simulink model "PX4_PID"  (R2023b)
settings: Solver=FixedStepAuto  StartTime=0.0  StopTime=inf  RelTol=1e-3  EnableMultiTasking=on
undefined symbols (not defined in the file): AUX, dev, pwm_output1
libraries: slpidlib x3, px4uORBlib x3, px4Sensorslib x2, px4lib x1, robotcorelib x1
settings Model: ExtModeTrigDuration=10  Creator=yamak  LastModifiedBy=sekiguchi
settings SolverCC: PositivePriorityOrder=on
settings OptimizationCC: EnhancedBackFolding=on  PassReuseOutputArgsAs=Individual arguments  ZeroExternalMemoryAtStartup=off  ZeroInternalMemoryAtStartup=off  MaxStackSize=64  OptimizeBlockOrder=speed  DifferentSizesBufferReuse=on  OptimizationCustomize=off  EfficientTunableParamExpr=on
settings DebuggingCC: ParameterTunabilityLossMsg=error
settings HardwareCC: ProdBitPerPointer=32  ProdBitPerSizeT=32  ProdBitPerPtrDiffT=32  ProdLargestAtomicInteger=Long  ProdLargestAtomicFloat=Double  ProdWordSize=32  ProdLongLongMode=on  ProdHWDeviceType=ARM Compatible->ARM Cortex
settings SFSimCC: MATLABDynamicMemAlloc=off  SimTargetLang=C++
settings RTWCC: Description=Embedded Coder  SystemTargetFile=ert.tlc  HardwareBoard=PX4 Pixhawk 6x  TLCOptions="-aInlineSetEventsForThisBaseRateFcn=TLC_FALSE -aSuppressMultiTaskScheduler=TLC_FALSE  -aRateBasedStepFcn=0"  TemplateMakefile=ert_default_tmf  Toolchain=GNU Tools for PX4 Autopilots  TargetLang=C++
settings CodeAppCC: ForceParamTrailComments=on  IgnoreCustomStorageClasses=off  OperatorAnnotations=on  SimulinkDataObjDesc=on  SFDataObjDesc=on  InsertBlockDesc=on
settings ERTTargetCC: ExtModeTransport=3  ExtModeStaticAlloc=on  ExtModeStaticAllocSize=1024  ExtModeMexFile=ext_xcp  ExtModeIntrfLevel=Level2 - Open

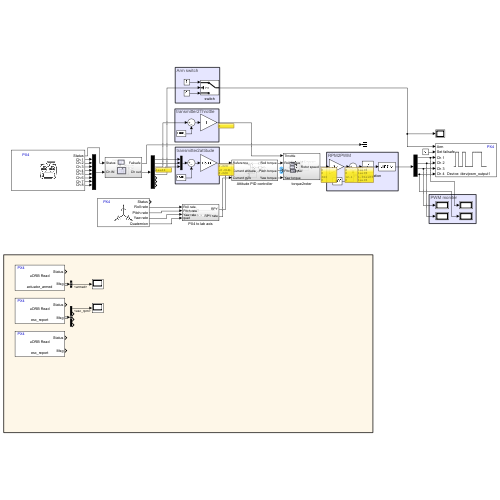
[thumbnail: Simulink's stored preview of the top-level diagram]
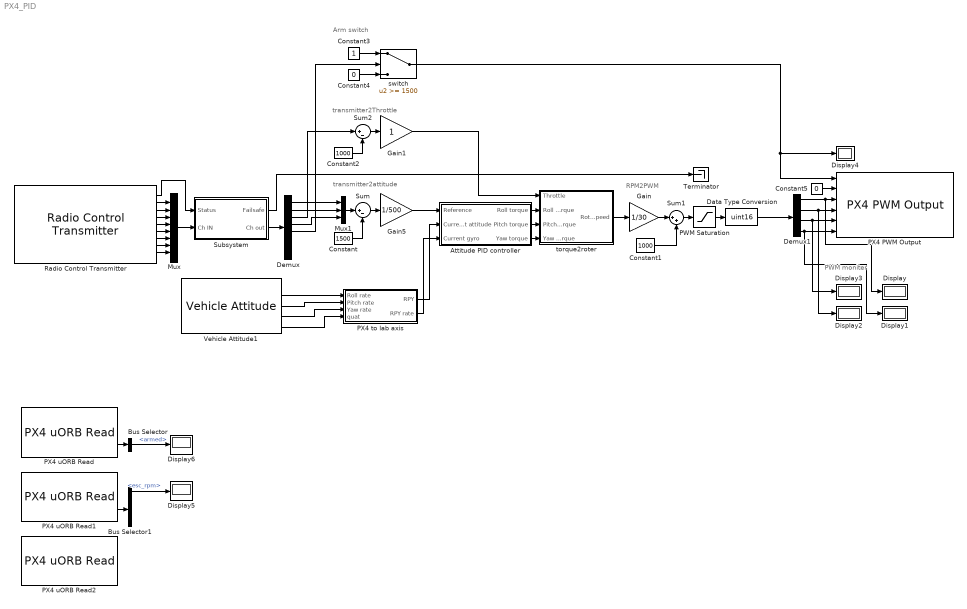
== system PX4_PID ==
  note: PWM moniter
  note: Arm switch
  note: transmitter2Throttle
  note: transmitter2attitude
  note: RPM2PWM
  Attitude PID controller : Subsystem
  Bus Selector : BusSelector  OutputSignals=armed
  Bus Selector1 : BusSelector  OutputSignals=esc_rpm,esc_voltage,esc_current,esc_temperature
  Constant : Constant  Value=1500
  Constant1 : Constant  Value=1000
  Constant2 : Constant  Value=1000
  Constant3 : Constant  OutDataTypeStr=boolean
  Constant4 : Constant  Value=0  OutDataTypeStr=boolean
  Constant5 : Constant  Value=0  OutDataTypeStr=boolean
  Data Type Conversion : DataTypeConversion  OutDataTypeStr=uint16  SaturateOnIntegerOverflow=off  RndMeth=Floor
  Demux : Demux  Outputs=8
  Demux1 : Demux
  Display{,1..6} (7 alike) : Display
  Gain : Gain  Gain=1/30
  Gain1 : Gain  OutDataTypeStr=double
  Gain5 : Gain  Gain=1/500  OutDataTypeStr=double
  Mux : Mux  Inputs=8
  Mux1 : Mux  Inputs=3
  PWM Saturation : Saturate  UpperLimit=2000  LowerLimit=1000
  PX4 PWM Output : px4lib/PX4 PWM Output  pwmDevice=AUX (/dev/pwm_output1)  pwmChannel1_=on  pwmChannel2_=on  pwmChannel3_=on  pwmChannel4_=on  pwmChannel5_=off  pwmChannel6_=off  pwmChannel7_=off  pwmChannel8_=off  forceTerminateFailsafe=off  outputErrorStatus=off
  PX4 to lab axis : Subsystem
  PX4 uORB Read : px4uORBlib/PX4 uORB Read  uORBTopic=actuator_armed  selectInstance=actuator_armed  SampleTime=0.001  BlockingMode=off  BlockTimeout=1e-3
  PX4 uORB Read1 : px4uORBlib/PX4 uORB Read  uORBTopic=esc_report  selectInstance=esc_report  SampleTime=0.001  BlockingMode=off  BlockTimeout=1e-3
  PX4 uORB Read2 : px4uORBlib/PX4 uORB Read  uORBTopic=esc_report  selectInstance=esc_report  SampleTime=0.001  BlockingMode=off  BlockTimeout=1e-3
  Radio Control Transmitter : px4Sensorslib/Radio Control Transmitter  channel1=on  channel2=on  channel3=on  channel4=on  channel5=on  channel6=on  channel7=on  channel8=on  channel_count=off  rssi=off  rc_input_source=off  timestamp_last_signal=off  time_stamp=off  sampleTime=1/250  BlockingMode=off  BlockTimeout=5
  Subsystem : Subsystem
  Sum : Sum  Inputs=|+-
  Sum1 : Sum  Inputs=|++
  Sum2 : Sum  Inputs=|+-
  Terminator : Terminator
  Vehicle Attitude1 : px4Sensorslib/Vehicle Attitude  rollRate=on  pitchRate=on  yawRate=on  quaternion=on  uorbTimeStamp=off  BlockingMode=off  BlockTimeout=0.001  sampleTime=1/250
  switch : Switch  Threshold=1500  OutDataTypeStr=boolean  SaturateOnIntegerOverflow=off  InputSameDT=off
  torque2roter : Subsystem
  wires:
  Vehicle Attitude1/5 -> PX4 to lab axis/4(quat)
  Constant/1 -> Sum/2
  Mux1/1 -> Sum/1
  Sum/1 -> Gain5/1
  Gain5/1 -> Attitude PID controller/1(Reference)
  Demux1/1 -> Display/1, PX4 PWM Output/3
  Demux1/2 -> PX4 PWM Output/4, Display2/1
  Demux1/3 -> PX4 PWM Output/5, Display3/1
  Demux1/4 -> Display1/1, PX4 PWM Output/6
  Data Type Conversion/1 -> Demux1/1
  Vehicle Attitude1/2 -> PX4 to lab axis/1(Roll rate)
  Vehicle Attitude1/3 -> PX4 to lab axis/2(Pitch rate)
  Vehicle Attitude1/4 -> PX4 to lab axis/3(Yaw rate)
  PWM Saturation/1 -> Data Type Conversion/1
  Sum1/1 -> PWM Saturation/1
  Constant1/1 -> Sum1/2
  Gain/1 -> Sum1/1
  torque2roter/1(Rotor speed) -> Gain/1
  PX4 to lab axis/1(RPY) -> Attitude PID controller/2(Current attitude)
  PX4 to lab axis/2(RPY rate) -> Attitude PID controller/3(Current gyro)
  Attitude PID controller/1(Roll torque) -> torque2roter/2(Roll torque)
  Attitude PID controller/2(Pitch torque) -> torque2roter/3(Pitch torque)
  Attitude PID controller/3(Yaw torque) -> torque2roter/4(Yaw torque)
  Sum2/1 -> Gain1/1
  Constant2/1 -> Sum2/2
  Gain1/1 -> torque2roter/1(Throttle)
  Radio Control Transmitter/1 -> Subsystem/1(Status)
  Radio Control Transmitter/9 -> Mux/8
  Radio Control Transmitter/2 -> Mux/1
  Radio Control Transmitter/3 -> Mux/2
  Radio Control Transmitter/4 -> Mux/3
  Radio Control Transmitter/5 -> Mux/4
  Radio Control Transmitter/6 -> Mux/5
  Radio Control Transmitter/7 -> Mux/6
  Radio Control Transmitter/8 -> Mux/7
  Mux/1 -> Subsystem/2(Ch IN)
  Subsystem/2(Ch out) -> Demux/1
  Demux/1 -> Mux1/1
  Demux/2 -> Mux1/2
  Demux/4 -> Mux1/3
  Demux/3 -> Sum2/1
  Constant3/1 -> switch/1
  Demux/5 -> switch/2
  Constant4/1 -> switch/3
  PX4 uORB Read/2 -> Bus Selector/1
  Bus Selector/1 -> Display6/1  "<armed>"
  switch/1 -> PX4 PWM Output/1, Display4/1
  Subsystem/1(Failsafe) -> Terminator/1
  PX4 uORB Read1/2 -> Bus Selector1/1
  Bus Selector1/1 -> Display5/1  "<esc_rpm>"
  Constant5/1 -> PX4 PWM Output/2

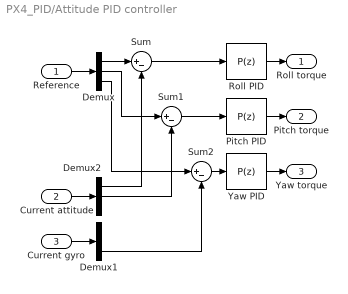
== system PX4_PID/Attitude PID controller ==
  Reference : Inport
  Current attitude : Inport  Port=2
  Current gyro : Inport  Port=3
  Demux : Demux  Outputs=3
  Demux1 : Demux  Outputs=3
  Demux2 : Demux  Outputs=3
  Pitch PID : slpidlib/PID Controller  Controller=P  Form=Parallel  TimeDomain=Discrete-time  UseExternalTs=off  SampleTime=-1  IntegratorMethod=Forward Euler  FilterMethod=Forward Euler  ControllerParametersSource=internal  P=1  I=1  UseKiTs=off  D=0  N=100  UseFilter=on  TunerSelectOption=Transfer Function Based (PID Tuner App)  InitialConditionSource=internal  InitialConditionForIntegrator=0  InitialConditionForFilter=0  DifferentiatorICPrevScaledInput=0  ExternalReset=none  TrackingMode=off  Kt=1  LimitOutput=off  SatLimitsSource=internal  UpperSaturationLimit=inf  LowerSaturationLimit=-inf  LinearizeAsGain=on  AntiWindupMode=none  Kb=1  LimitIntegrator=off  UpperIntegratorSaturationLimit=inf  LowerIntegratorSaturationLimit=-inf  POutMin=[]  POutMax=[]  IOutMin=[]  IOutMax=[]  DOutMin=[]  DOutMax=[]  NOutMin=[]  NOutMax=[]  SumOutMin=[]  SumOutMax=[]  SaturationOutMin=[]  SaturationOutMax=[]  PParamMin=[]  PParamMax=[]  IParamMin=[]  IParamMax=[]  DParamMin=[]  DParamMax=[]  NParamMin=[]  NParamMax=[]  KbParamMin=[]  KbParamMax=[]  KtParamMin=[]  KtParamMax=[]  KbOutMin=[]  KbOutMax=[]  KtOutMin=[]  KtOutMax=[]  IntegratorOutMin=[]  IntegratorOutMax=[]  FilterOutMin=[]  FilterOutMax=[]  SumI1OutMin=[]  SumI1OutMax=[]  SumI2OutMin=[]  SumI2OutMax=[]  SumI3OutMin=[]  SumI3OutMax=[]  SumI4OutMin=[]  SumI4OutMax=[]  SumDOutMin=[]  SumDOutMax=[]  DifferentiatorOutMin=[]  DifferentiatorOutMax=[]  FilterDiffOutCoefMin=[]  FilterDiffOutCoefMax=[]  ReciprocalOutMin=[]  ReciprocalOutMax=[]  SumDenOutMin=[]  SumDenOutMax=[]  SumNumOutMin=[]  SumNumOutMax=[]  DivideOutMin=[]  DivideOutMax=[]  UdiffTsProdOutMin=[]  UdiffTsProdOutMax=[]  NTsProdOutMin=[]  NTsProdOutMax=[]  UintegralTsProdOutMin=[]  UintegralTsProdOutMax=[]  UngainTsProdOutMin=[]  UngainTsProdOutMax=[]  ClampingZeroOutDataTypeStr=Inherit: Inherit via back propagation  ClampingZeroOutMin=[]  ClampingZeroOutMax=[]  FilterDenConstantOutDataTypeStr=Inherit: Inherit via back propagation  FilterDenConstantOutMin=[]  FilterDenConstantOutMax=[]  PCopyOutDataTypeStr=Inherit: Inherit via back propagation  PCopyOutMin=[]  PCopyOutMax=[]  NCopyOutDataTypeStr=Inherit: Inherit via back propagation  NCopyOutMin=[]  NCopyOutMax=[]  IntegratorContinuousStateAttributes=''  IntegratorStateMustResolveToSignalObject=off  IntegratorRTWStateStorageClass=Auto  FilterContinuousStateAttributes=''  FilterStateMustResolveToSignalObject=off  FilterRTWStateStorageClass=Auto  ParallelPVariant=InternalParameters  IdealPVariant=Disabled  IVariant=Disabled  DVariant=Disabled  IntegratorVariant=Disabled  SatVariant=Disabled  AWVariant=Disabled  PCopyVariant=Disabled  TRVariant=Disabled  FdbkBlocksVariant=Forward  IdealPFdbkVariant=Disabled  SatFdbkVariant=Disabled  DerivativeFilterVariant=Disabled  NVariant=Disabled  NCopyVariant=Disabled_SignalSpec  FilterICVariant=Disabled  IntegratorICVariant=Disabled  ExternalResetVariant=Disabled  TRSumVariant=Passthrough  SumFdbkVariant=Disabled  SumVariant=Passthrough_P  TsampFilterVariant=InternalTs  TsampNgainVariant=Passthrough  TsampIntegralVariant=Disabled_SignalSpec  ExternalSaturationOutDataTypeStr=Inherit: Same as second input
  Roll PID : slpidlib/PID Controller  Controller=P  Form=Parallel  TimeDomain=Discrete-time  UseExternalTs=off  SampleTime=-1  IntegratorMethod=Forward Euler  FilterMethod=Forward Euler  ControllerParametersSource=internal  P=1  I=1  UseKiTs=off  D=0  N=100  UseFilter=on  TunerSelectOption=Transfer Function Based (PID Tuner App)  InitialConditionSource=internal  InitialConditionForIntegrator=0  InitialConditionForFilter=0  DifferentiatorICPrevScaledInput=0  ExternalReset=none  TrackingMode=off  Kt=1  LimitOutput=off  SatLimitsSource=internal  UpperSaturationLimit=inf  LowerSaturationLimit=-inf  LinearizeAsGain=on  AntiWindupMode=none  Kb=1  LimitIntegrator=off  UpperIntegratorSaturationLimit=inf  LowerIntegratorSaturationLimit=-inf  POutMin=[]  POutMax=[]  IOutMin=[]  IOutMax=[]  DOutMin=[]  DOutMax=[]  NOutMin=[]  NOutMax=[]  SumOutMin=[]  SumOutMax=[]  SaturationOutMin=[]  SaturationOutMax=[]  PParamMin=[]  PParamMax=[]  IParamMin=[]  IParamMax=[]  DParamMin=[]  DParamMax=[]  NParamMin=[]  NParamMax=[]  KbParamMin=[]  KbParamMax=[]  KtParamMin=[]  KtParamMax=[]  KbOutMin=[]  KbOutMax=[]  KtOutMin=[]  KtOutMax=[]  IntegratorOutMin=[]  IntegratorOutMax=[]  FilterOutMin=[]  FilterOutMax=[]  SumI1OutMin=[]  SumI1OutMax=[]  SumI2OutMin=[]  SumI2OutMax=[]  SumI3OutMin=[]  SumI3OutMax=[]  SumI4OutMin=[]  SumI4OutMax=[]  SumDOutMin=[]  SumDOutMax=[]  DifferentiatorOutMin=[]  DifferentiatorOutMax=[]  FilterDiffOutCoefMin=[]  FilterDiffOutCoefMax=[]  ReciprocalOutMin=[]  ReciprocalOutMax=[]  SumDenOutMin=[]  SumDenOutMax=[]  SumNumOutMin=[]  SumNumOutMax=[]  DivideOutMin=[]  DivideOutMax=[]  UdiffTsProdOutMin=[]  UdiffTsProdOutMax=[]  NTsProdOutMin=[]  NTsProdOutMax=[]  UintegralTsProdOutMin=[]  UintegralTsProdOutMax=[]  UngainTsProdOutMin=[]  UngainTsProdOutMax=[]  ClampingZeroOutDataTypeStr=Inherit: Inherit via back propagation  ClampingZeroOutMin=[]  ClampingZeroOutMax=[]  FilterDenConstantOutDataTypeStr=Inherit: Inherit via back propagation  FilterDenConstantOutMin=[]  FilterDenConstantOutMax=[]  PCopyOutDataTypeStr=Inherit: Inherit via back propagation  PCopyOutMin=[]  PCopyOutMax=[]  NCopyOutDataTypeStr=Inherit: Inherit via back propagation  NCopyOutMin=[]  NCopyOutMax=[]  IntegratorContinuousStateAttributes=''  IntegratorStateMustResolveToSignalObject=off  IntegratorRTWStateStorageClass=Auto  FilterContinuousStateAttributes=''  FilterStateMustResolveToSignalObject=off  FilterRTWStateStorageClass=Auto  ParallelPVariant=InternalParameters  IdealPVariant=Disabled  IVariant=Disabled  DVariant=Disabled  IntegratorVariant=Disabled  SatVariant=Disabled  AWVariant=Disabled  PCopyVariant=Disabled  TRVariant=Disabled  FdbkBlocksVariant=Forward  IdealPFdbkVariant=Disabled  SatFdbkVariant=Disabled  DerivativeFilterVariant=Disabled  NVariant=Disabled  NCopyVariant=Disabled_SignalSpec  FilterICVariant=Disabled  IntegratorICVariant=Disabled  ExternalResetVariant=Disabled  TRSumVariant=Passthrough  SumFdbkVariant=Disabled  SumVariant=Passthrough_P  TsampFilterVariant=InternalTs  TsampNgainVariant=Passthrough  TsampIntegralVariant=Disabled_SignalSpec  ExternalSaturationOutDataTypeStr=Inherit: Same as second input
  Sum : Sum  Inputs=|+-
  Sum1 : Sum  Inputs=|+-
  Sum2 : Sum  Inputs=|+-
  Yaw PID : slpidlib/PID Controller  Controller=P  Form=Parallel  TimeDomain=Discrete-time  UseExternalTs=off  SampleTime=-1  IntegratorMethod=Forward Euler  FilterMethod=Forward Euler  ControllerParametersSource=internal  P=1  I=1  UseKiTs=off  D=0  N=100  UseFilter=on  TunerSelectOption=Transfer Function Based (PID Tuner App)  InitialConditionSource=internal  InitialConditionForIntegrator=0  InitialConditionForFilter=0  DifferentiatorICPrevScaledInput=0  ExternalReset=none  TrackingMode=off  Kt=1  LimitOutput=off  SatLimitsSource=internal  UpperSaturationLimit=inf  LowerSaturationLimit=-inf  LinearizeAsGain=on  AntiWindupMode=none  Kb=1  LimitIntegrator=off  UpperIntegratorSaturationLimit=inf  LowerIntegratorSaturationLimit=-inf  POutMin=[]  POutMax=[]  IOutMin=[]  IOutMax=[]  DOutMin=[]  DOutMax=[]  NOutMin=[]  NOutMax=[]  SumOutMin=[]  SumOutMax=[]  SaturationOutMin=[]  SaturationOutMax=[]  PParamMin=[]  PParamMax=[]  IParamMin=[]  IParamMax=[]  DParamMin=[]  DParamMax=[]  NParamMin=[]  NParamMax=[]  KbParamMin=[]  KbParamMax=[]  KtParamMin=[]  KtParamMax=[]  KbOutMin=[]  KbOutMax=[]  KtOutMin=[]  KtOutMax=[]  IntegratorOutMin=[]  IntegratorOutMax=[]  FilterOutMin=[]  FilterOutMax=[]  SumI1OutMin=[]  SumI1OutMax=[]  SumI2OutMin=[]  SumI2OutMax=[]  SumI3OutMin=[]  SumI3OutMax=[]  SumI4OutMin=[]  SumI4OutMax=[]  SumDOutMin=[]  SumDOutMax=[]  DifferentiatorOutMin=[]  DifferentiatorOutMax=[]  FilterDiffOutCoefMin=[]  FilterDiffOutCoefMax=[]  ReciprocalOutMin=[]  ReciprocalOutMax=[]  SumDenOutMin=[]  SumDenOutMax=[]  SumNumOutMin=[]  SumNumOutMax=[]  DivideOutMin=[]  DivideOutMax=[]  UdiffTsProdOutMin=[]  UdiffTsProdOutMax=[]  NTsProdOutMin=[]  NTsProdOutMax=[]  UintegralTsProdOutMin=[]  UintegralTsProdOutMax=[]  UngainTsProdOutMin=[]  UngainTsProdOutMax=[]  ClampingZeroOutDataTypeStr=Inherit: Inherit via back propagation  ClampingZeroOutMin=[]  ClampingZeroOutMax=[]  FilterDenConstantOutDataTypeStr=Inherit: Inherit via back propagation  FilterDenConstantOutMin=[]  FilterDenConstantOutMax=[]  PCopyOutDataTypeStr=Inherit: Inherit via back propagation  PCopyOutMin=[]  PCopyOutMax=[]  NCopyOutDataTypeStr=Inherit: Inherit via back propagation  NCopyOutMin=[]  NCopyOutMax=[]  IntegratorContinuousStateAttributes=''  IntegratorStateMustResolveToSignalObject=off  IntegratorRTWStateStorageClass=Auto  FilterContinuousStateAttributes=''  FilterStateMustResolveToSignalObject=off  FilterRTWStateStorageClass=Auto  ParallelPVariant=InternalParameters  IdealPVariant=Disabled  IVariant=Disabled  DVariant=Disabled  IntegratorVariant=Disabled  SatVariant=Disabled  AWVariant=Disabled  PCopyVariant=Disabled  TRVariant=Disabled  FdbkBlocksVariant=Forward  IdealPFdbkVariant=Disabled  SatFdbkVariant=Disabled  DerivativeFilterVariant=Disabled  NVariant=Disabled  NCopyVariant=Disabled_SignalSpec  FilterICVariant=Disabled  IntegratorICVariant=Disabled  ExternalResetVariant=Disabled  TRSumVariant=Passthrough  SumFdbkVariant=Disabled  SumVariant=Passthrough_P  TsampFilterVariant=InternalTs  TsampNgainVariant=Passthrough  TsampIntegralVariant=Disabled_SignalSpec  ExternalSaturationOutDataTypeStr=Inherit: Same as second input
  Roll torque : Outport
  Pitch torque : Outport  Port=2
  Yaw torque : Outport  Port=3
  wires:
  Roll PID/1 -> Roll torque/1
  Reference/1 -> Demux/1
  Demux/1 -> Sum/1
  Demux/2 -> Sum1/1
  Current gyro/1 -> Demux1/1
  Demux/3 -> Sum2/1
  Sum/1 -> Roll PID/1
  Demux2/1 -> Sum/2
  Sum1/1 -> Pitch PID/1
  Demux2/2 -> Sum1/2
  Sum2/1 -> Yaw PID/1
  Demux1/3 -> Sum2/2
  Current attitude/1 -> Demux2/1
  Pitch PID/1 -> Pitch torque/1
  Yaw PID/1 -> Yaw torque/1

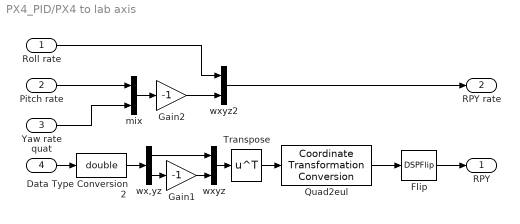
== system PX4_PID/PX4 to lab axis ==
  Roll rate : Inport
  Pitch rate : Inport  Port=2
  Yaw rate : Inport  Port=3
  quat : Inport  Port=4
  Data Type Conversion2 : DataTypeConversion  OutDataTypeStr=double  SaturateOnIntegerOverflow=off  RndMeth=Floor
  Flip : DSPFlip
  Gain1 : Gain  Gain=-1
  Gain2 : Gain  Gain=-1
  Quad2eul : robotcorelib/Coordinate Transformation Conversion  InputRepresentation=Quaternion  InputEulerSequence=ZYX  ShowTrVecInputPort=on  OutputRepresentation=Euler Angles  OutputEulerSequence=ZYX  ShowTrVecOutputPort=on  SimulateUsing=Interpreted execution
      settings: LibrarySourceBlock=uavutilslib/Coordinate Transformation Conversion
  Transpose : Math  Operator=transpose
  mix : Mux  Inputs=2
  wx,yz : Demux  Outputs=2
  wxyz : Mux  Inputs=2
  wxyz2 : Mux  Inputs=2
  RPY : Outport
  RPY rate : Outport  Port=2
  wires:
  quat/1 -> Data Type Conversion2/1
  Data Type Conversion2/1 -> wx,yz/1
  wx,yz/2 -> Gain1/1
  wx,yz/1 -> wxyz/1
  Gain1/1 -> wxyz/2
  wxyz/1 -> Transpose/1
  Quad2eul/1 -> Flip/1
  Transpose/1 -> Quad2eul/1
  Flip/1 -> RPY/1
  Pitch rate/1 -> mix/1
  Yaw rate/1 -> mix/2
  mix/1 -> Gain2/1
  Gain2/1 -> wxyz2/2
  Roll rate/1 -> wxyz2/1
  wxyz2/1 -> RPY rate/1

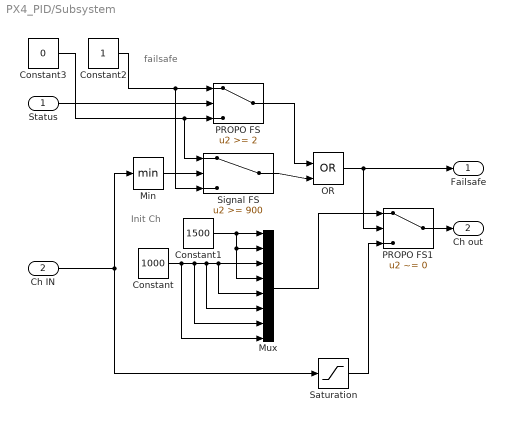
== system PX4_PID/Subsystem ==
  note: Init Ch
  note: failsafe
  Status : Inport
  Ch IN : Inport  Port=2
  Constant : Constant  Value=1000
  Constant1 : Constant  Value=1500
  Constant2 : Constant  OutDataTypeStr=boolean
  Constant3 : Constant  Value=0  OutDataTypeStr=boolean
  Min : MinMax
  Mux : Mux  Inputs=8
  OR : Logic  Operator=OR  IconShape=distinctive  AllPortsSameDT=off  OutDataTypeStr=boolean
  PROPO FS : Switch  Threshold=2  OutDataTypeStr=boolean  SaturateOnIntegerOverflow=off  InputSameDT=off
  PROPO FS1 : Switch  Criteria=u2 ~= 0  Threshold=2  SaturateOnIntegerOverflow=off  InputSameDT=off
  Saturation : Saturate  UpperLimit=2000  LowerLimit=1000
  Signal FS : Switch  Threshold=900  OutDataTypeStr=boolean  SaturateOnIntegerOverflow=off  InputSameDT=off
  Failsafe : Outport
  Ch out : Outport  Port=2
  wires:
  Constant1/1 -> Mux/1, Mux/4, Mux/2
  Constant/1 -> Mux/8, Mux/7, Mux/6, Mux/5, Mux/3
  Constant3/1 -> Signal FS/1, PROPO FS/3
  PROPO FS/1 -> OR/1
  Ch IN/1 -> Min/1, Saturation/1
  Mux/1 -> PROPO FS1/1
  PROPO FS1/1 -> Ch out/1
  OR/1 -> Failsafe/1, PROPO FS1/2
  Status/1 -> PROPO FS/2
  Min/1 -> Signal FS/2
  Constant2/1 -> PROPO FS/1, Signal FS/3
  Signal FS/1 -> OR/2
  Saturation/1 -> PROPO FS1/3

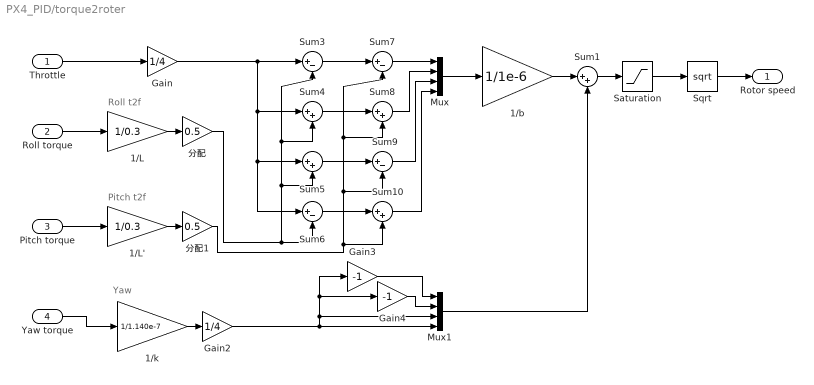
== system PX4_PID/torque2roter ==
  note: Pitch t2f
  note: Roll t2f
  note: Yaw
  Throttle : Inport
  Roll torque : Inport  Port=2
  Pitch torque : Inport  Port=3
  Yaw torque : Inport  Port=4
  1/L : Gain  Gain=1/0.3
  1/L' : Gain  Gain=1/0.3
  1/b : Gain  Gain=1/1e-6
  1/k : Gain  Gain=1/1.140e-7
  Gain : Gain  Gain=1/4
  Gain2 : Gain  Gain=1/4
  Gain3 : Gain  Gain=-1
  Gain4 : Gain  Gain=-1
  Mux : Mux
  Mux1 : Mux
  Saturation : Saturate  UpperLimit=inf  LowerLimit=0
  Sqrt : Sqrt
  Sum{1,4..5,8,10} (5 alike) : Sum  Inputs=|++
  Sum{3,6..7,9} (4 alike) : Sum  Inputs=|+-
  分配 : Gain  Gain=0.5
  分配1 : Gain  Gain=0.5
  Rotor speed : Outport
  wires:
  Gain/1 -> Sum6/1, Sum5/1, Sum4/1, Sum3/1
  Sum3/1 -> Sum7/1
  Sum4/1 -> Sum8/1
  Sum5/1 -> Sum9/1
  Sum6/1 -> Sum10/1
  Mux/1 -> 1/b/1
  分配1/1 -> Sum10/2, Sum9/2, Sum8/2, Sum7/2
  Pitch torque/1 -> 1/L'/1
  分配/1 -> Sum3/2, Sum4/2, Sum5/2, Sum6/2
  Throttle/1 -> Gain/1
  Roll torque/1 -> 1/L/1
  Sum7/1 -> Mux/1
  Sum8/1 -> Mux/2
  Sum9/1 -> Mux/3
  Sum10/1 -> Mux/4
  Yaw torque/1 -> 1/k/1
  1/L/1 -> 分配/1
  1/L'/1 -> 分配1/1
  1/k/1 -> Gain2/1
  Gain3/1 -> Mux1/1
  Gain4/1 -> Mux1/2
  Mux1/1 -> Sum1/2
  Gain2/1 -> Gain4/1, Gain3/1, Mux1/3, Mux1/4
  1/b/1 -> Sum1/1
  Sqrt/1 -> Rotor speed/1
  Sum1/1 -> Saturation/1
  Saturation/1 -> Sqrt/1
